simulink model "self_triggered_mpc_simulation_1"  (R2023a)
settings: Solver=VariableStepAuto  StartTime=0.0  StopTime=1  RelTol=1e-3
values from neighbouring files (symbols this model uses):
  param = param.param    [autometica_mpc.m]    (also in cost_cal.m = param_setup(); main.m = param_setup(); para.m = struct; param.mat = )
settings Model: Creator=김준수  LastModifiedBy=김준수

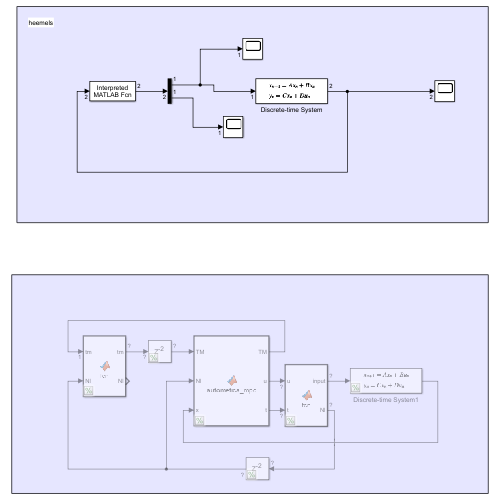
[thumbnail: Simulink's stored preview of the top-level diagram]
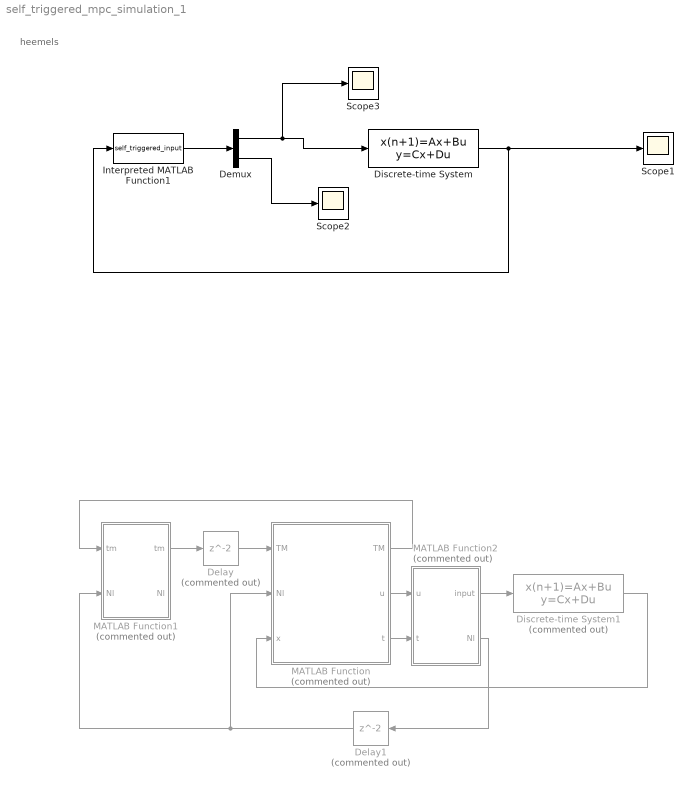
== system self_triggered_mpc_simulation_1 ==
  note: heemels
  Delay : Delay  Commented=on
  Delay1 : Delay  Commented=on
  Demux : Demux  Outputs=2
  Discrete-time System : DiscreteStateSpace  A=param.A  B=param.B  C=eye(param.nx)  D=zeros(param.nx,1)  InitialCondition=param.x0
  Discrete-time System1 : DiscreteStateSpace  Commented=on  A=param.A  B=param.B  C=eye(param.nx)  D=zeros(param.nx,1)  InitialCondition=param.x0
  Interpreted MATLAB Function1 : MATLABFcn  MATLABFcn=self_triggered_input  OutputDimensions=param.nu+1  Output1D=off
  MATLAB Function : MATLAB Function  Commented=on  TreatAsAtomicUnit=on
  MATLAB Function1 : MATLAB Function  Commented=on  TreatAsAtomicUnit=on
  MATLAB Function2 : MATLAB Function  Commented=on  TreatAsAtomicUnit=on
  Scope1 : Scope
  Scope2 : Scope
  Scope3 : Scope
  wires:
  Discrete-time System/1 -> Scope1/1, Interpreted MATLAB Function1/1
  Interpreted MATLAB Function1/1 -> Demux/1
  Demux/1 -> Scope3/1, Discrete-time System/1
  Demux/2 -> Scope2/1
  Discrete-time System1/1 -> MATLAB Function/3(x)
  MATLAB Function/1(TM) -> MATLAB Function1/1("tm ")
  Delay/1 -> MATLAB Function/1("TM ")
  MATLAB Function1/1(tm) -> Delay/1
  MATLAB Function/2(u) -> MATLAB Function2/1(u)
  MATLAB Function/3(t) -> MATLAB Function2/2(t)
  MATLAB Function2/1(input) -> Discrete-time System1/1
  MATLAB Function2/2(Nl) -> Delay1/1
  Delay1/1 -> MATLAB Function/2(Nl), MATLAB Function1/2("Nl ")

== matlab function self_triggered_mpc_simulation_1/MATLAB Function1 ==
  data: tm input; tm output; Nl output; Nl input
function [tm , Nl] = fcn(tm, Nl)

y = u;

== matlab function self_triggered_mpc_simulation_1/MATLAB Function ==
  data: TM output; u output; t output; TM input; Nl input; x input
function [TM, u, t] = autometica_mpc(TM, Nl, x)

    coder.extrinsic("optimconstr", "optimproblem", "optimvar");
%==========================================================================
 %parameter setting
    param = load("param.mat");
    param = param.param;


%==========================================================================
    %implement autometica vesion
    prob = optimproblem;
    x0 = optimvar('x0', param.nx);
    x = optimvar('x', param.nx,N);
    u0 = optimvar('x', param.nu);
    u = optimvar('u',param.nu, N-1);
    
    cost_function =x0'*param.Q*x0+u0*param.R*u0;
    for i=1:param.N-1
        cost_function = cost_function + x(:,i)'*param.Q*x(:,i)  + u(:,i)'*param.Q*u(:,i); % terminal cost 설정해야 됨
    end
    prob.Objective = cost_function;
    
%==========================================================================
% model constraints

    model_constr = optimconstr((param.N)+1);
    model_constr(1) = x(:,1) == param.A*x0 + param.B*u0;
    for i=1:param.N-1
        model_constr(i+1) = x(:,i+1) == param.A*x(:,i) + param.B*u(:,i);
    end
    model_constr((param.N)+1) = x0 == x;
    prob.Constraints.model_constr = model_constr;
    
%==========================================================================
%terminal set constraints
    constT = optimconstr(30,Tset+1);
       
    LL = param.tildeF - param.tildeG*param.tildeK;
    PHI = (param.tildeA - param.tildeB*param.tildeK);
    PSI = []
    for i= 1:Tset
        constT(:,i) = LL*(param.phi^(i))*x(:,M+Nl)<=[1; 1;1; 1;1; 1;];
    end
    constT(1:param.NumOfConstr,Tset+1) = (param.F-param.G*param.K)*x(:,M+Nl)<=1;
    prob.Constraints.ConstT = constT;
%==========================================================================
% triggering constraints
    triggering_constr = optimconstr(param.N);
    triggering_constr(1) = u0 == u(:,1);
    for i = 1:param.N-2
        triggering_constr(i+1) = u(:,i)==u(:,i+1);
    end

== matlab function self_triggered_mpc_simulation_1/MATLAB Function2 ==
  data: u input; input output; t input; Nl output
function [input, Nl] = fcn(u,t)
param = loda('param.mat');
param = param.param;
Nl = 2*param.M - t;

y = u;
